simulink model "userdefined_funtion_test"  (R2014b)
settings: Solver=ode45  StartTime=0.0  StopTime=10.0  RelTol=1e-3
settings Model: Creator=brownaa  LastModifiedBy=brownaa

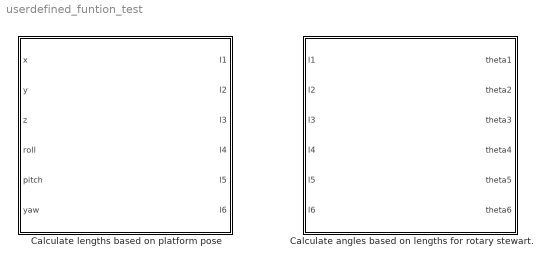
== system userdefined_funtion_test ==
  " Calculate angles based on lengths for rotary stewart." : MATLAB Function  TreatAsAtomicUnit=on
  Calculate lengths based on platform pose : MATLAB Function  TreatAsAtomicUnit=on

== matlab function userdefined_funtion_test/Calculate lengths based on platform pose ==
  data: x input; y input; z input; roll input; pitch input; yaw input; l1 output; l2 output; l3 output; l4 output; l5 output; l6 output
function [l1,l2,l3,l4,l5,l6] = fcn(x,y,z,roll,pitch,yaw)
%#codegen

l1=0;
l2=0;
l3=0;
l4=0;
l5=0;
l6=0;
end

== matlab function userdefined_funtion_test/ Calculate angles based on lengths for rotary stewart. ==
  data: l1 input; l2 input; l3 input; l4 input; l5 input; l6 input; theta1 output; theta2 output; theta3 output; theta4 output; theta5 output; theta6 output
function [theta1,theta2,theta3,theta4,theta5,theta6] = fcn(l1,l2,l3,l4,l5,l6)
%#codegen

l1=0;
l2=0;
l3=0;
l4=0;
l5=0;
l6=0;
end
